simulink model "middle_ear_filter"  (R2020b)
settings: Solver=FixedStepDiscrete  StartTime=0.0  StopTime=stopTime  RelTol=1e-3
InitFcn:
  | initCallback
StopFcn:
  | stopCallback
values from neighbouring files (symbols this model uses):
  MEcoeffs = [m14*m11 m15*m11 m16*m11 1 m12*m11 m13*m11; m24*m21 m25*m21 m26*m21 1 m22*m21 m23*m21; m34*m31 m35*m31 m36*m31 1 m32*m31 m33*m31]    [mef_parameters.m]    (also in middle_ear_filter_parameter.m)
  MEscale = 1/megainmax    (= 0.5)    [mef_parameters.m]    (also in middle_ear_filter_parameter.m)
undefined symbols (not defined in the file or in its folder): mp
settings Model: Creator=Ross  LastModifiedBy=conno
settings DataIOCC: ReturnWorkspaceOutputs=off
settings OptimizationCC: BlockReduction=off  ConditionallyExecuteInputs=off  DefaultParameterBehavior=Inlined
settings DebuggingCC: ReadBeforeWriteMsg=DisableAll  WriteAfterWriteMsg=DisableAll  WriteAfterReadMsg=DisableAll  AlgebraicLoopMsg=error  MultiTaskDSMMsg=none  SingleTaskRateTransMsg=error  PregeneratedLibrarySubsystemCodeDiagnostic=none  ArithmeticOperatorsInVariantConditions=warning
settings HardwareCC: ProdBitPerPointer=32  ProdBitPerSizeT=32  ProdBitPerPtrDiffT=32  ProdLargestAtomicFloat=None  ProdIntDivRoundTo=Undefined  ProdEndianess=Unspecified  ProdWordSize=32  ProdHWDeviceType=ASIC/FPGA->ASIC/FPGA  TargetBitPerPointer=64  TargetBitPerSizeT=64  TargetBitPerPtrDiffT=64  TargetLongLongMode=on  TargetIntDivRoundTo=Zero  TargetEndianess=LittleEndian  TargetWordSize=64  TargetHWDeviceType=Custom Processor->MATLAB Host Computer  ProdEqTarget=off
settings ModelReferenceCC: UpdateModelReferenceTargets=IfOutOfDate
settings SFSimCC: SFSimEcho=off  SimUseLocalCustomCode=off  CustomCodeUndefinedFunction=UseInterfaceOnly
settings RTWCC: RTWUseLocalCustomCode=off

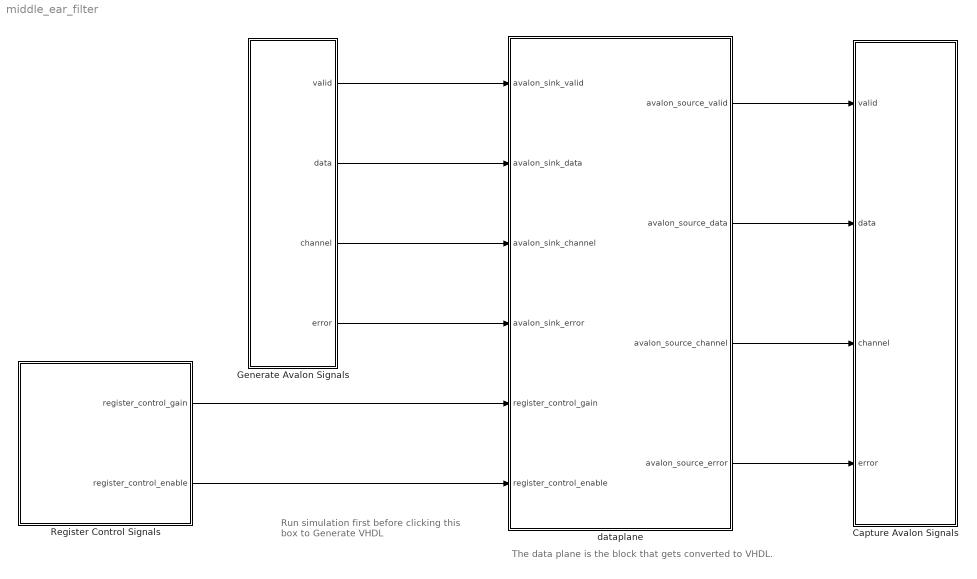
== system middle_ear_filter ==
  note: The data plane is the block that gets converted to VHDL.
  note: Run simulation first
      | before clicking this box to
      | Generate VHDL
  Capture Avalon Signals : Subsystem
  Generate Avalon Signals : Subsystem
  Register Control Signals : Subsystem
  dataplane : Subsystem  TreatAsAtomicUnit=on
  wires:
  Generate Avalon Signals/2(data) -> dataplane/2(avalon_sink_data)
  Generate Avalon Signals/1(valid) -> dataplane/1(avalon_sink_valid)
  Generate Avalon Signals/3(channel) -> dataplane/3(avalon_sink_channel)
  Generate Avalon Signals/4(error) -> dataplane/4(avalon_sink_error)
  dataplane/2(avalon_source_data) -> Capture Avalon Signals/2(data)
  dataplane/1(avalon_source_valid) -> Capture Avalon Signals/1(valid)
  dataplane/3(avalon_source_channel) -> Capture Avalon Signals/3(channel)
  dataplane/4(avalon_source_error) -> Capture Avalon Signals/4(error)
  Register Control Signals/1(register_control_gain) -> dataplane/5(register_control_gain)
  Register Control Signals/2(register_control_enable) -> dataplane/6(register_control_enable)

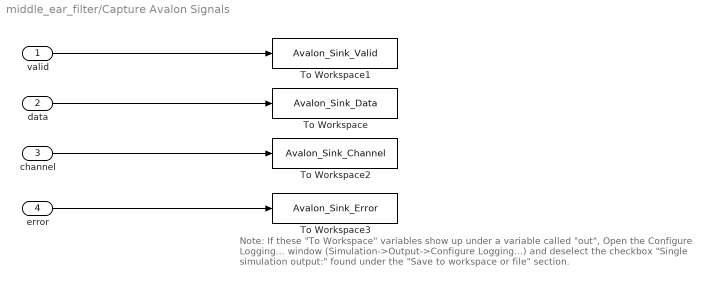
== system middle_ear_filter/Capture Avalon Signals ==
  note: Note:  If these "To Workspace" variables show up under a variable called "out",
      | Open the Configure Logging... window (Simulation->Output->Configure Logging...)
      | and deselect the checkbox "Single simulation output:" found under the "Save to workspace or file" section.
  valid : Inport
  data : Inport  Port=2
  channel : Inport  Port=3
  error : Inport  Port=4
  To Workspace : ToWorkspace  VariableName=Avalon_Sink_Data  SaveFormat=Timeseries  SampleTime=-1
  To Workspace1 : ToWorkspace  VariableName=Avalon_Sink_Valid  SaveFormat=Timeseries  SampleTime=-1
  To Workspace2 : ToWorkspace  VariableName=Avalon_Sink_Channel  SaveFormat=Timeseries  SampleTime=-1
  To Workspace3 : ToWorkspace  VariableName=Avalon_Sink_Error  SaveFormat=Timeseries  SampleTime=-1
  wires:
  data/1 -> To Workspace/1
  valid/1 -> To Workspace1/1
  error/1 -> To Workspace3/1
  channel/1 -> To Workspace2/1

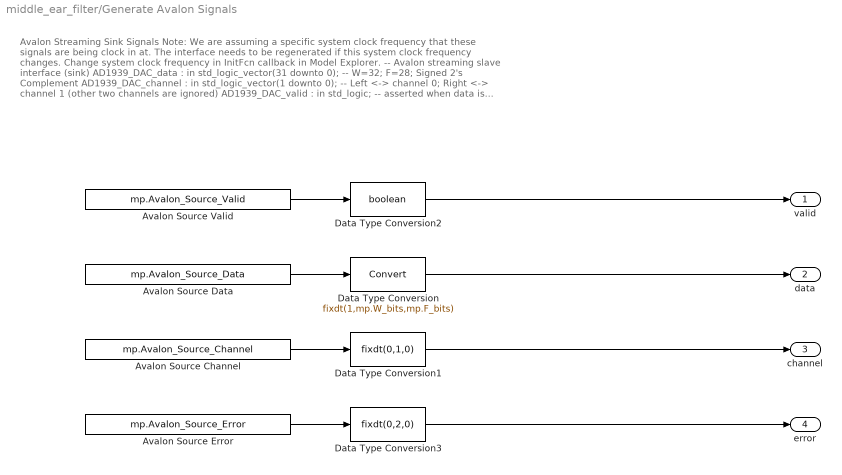
== system middle_ear_filter/Generate Avalon Signals ==
  note: Avalon Streaming Sink Signals
      | Note: We are assuming a specific system clock frequency that these signals are being clock in at.
      | The interface needs to be regenerated if this system clock frequency changes. Change system clock frequency in InitFcn callback in Model Explorer.
      |
      | -- Avalon streaming slave interface (sink)
      | AD1939_DAC_data : in std_logic_vector(31 downto 0); -- W=32; F=28; Signed 2's Complement
      | AD1939_DAC_channel : in std_logic_vector(1 downto 0); -- Left <-> channel 0; Right <-> channel 1 (other two channels are ignored)
      | AD1939_DAC_valid : in std_logic; -- asserted when data is valid
      | AD1939_DAC_error : in std_logic_vector(1 downto 0) -- error channel is ignored, assumed to be error free at this point
      |
      | For more information on the data-channel-valid protocol, s ee chapter 5 in Intel's Avalon Interfaced Specification (p. 40) at https://www.intel.com/content/dam/www/programmable/us/en/pdfs/literature/manual/mnl_avalon_spec.pdf
  Avalon Source Channel : FromWorkspace  VariableName=mp.Avalon_Source_Channel  OutDataTypeStr=double  SampleTime=mp.Ts_sim
  "Avalon Source Data " : FromWorkspace  VariableName=mp.Avalon_Source_Data  OutDataTypeStr=double  SampleTime=mp.Ts_sim
  Avalon Source Error : FromWorkspace  VariableName=mp.Avalon_Source_Error  OutDataTypeStr=double  SampleTime=mp.Ts_sim
  Avalon Source Valid : FromWorkspace  VariableName=mp.Avalon_Source_Valid  OutDataTypeStr=double  SampleTime=mp.Ts_sim
  Data Type Conversion : DataTypeConversion  OutDataTypeStr=fixdt(1,mp.W_bits,mp.F_bits)
  Data Type Conversion1 : DataTypeConversion  OutDataTypeStr=fixdt(0,1,0)
  Data Type Conversion2 : DataTypeConversion  OutDataTypeStr=boolean
  Data Type Conversion3 : DataTypeConversion  OutDataTypeStr=fixdt(0,2,0)
  valid : Outport  VectorParamsAs1DForOutWhenUnconnected=off
  data : Outport  Port=2  VectorParamsAs1DForOutWhenUnconnected=off
  channel : Outport  Port=3  VectorParamsAs1DForOutWhenUnconnected=off
  error : Outport  Port=4  VectorParamsAs1DForOutWhenUnconnected=off
  wires:
  Data Type Conversion1/1 -> channel/1
  Data Type Conversion2/1 -> valid/1
  Avalon Source Error/1 -> Data Type Conversion3/1
  Data Type Conversion/1 -> data/1
  Avalon Source Valid/1 -> Data Type Conversion2/1
  Data Type Conversion3/1 -> error/1
  Avalon Source Channel/1 -> Data Type Conversion1/1
  "Avalon Source Data "/1 -> Data Type Conversion/1

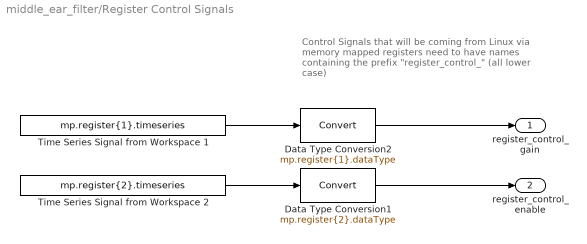
== system middle_ear_filter/Register Control Signals ==
  note: Control Signals that will be coming from Linux via
      | memory mapped registers need to have names
      | containing the prefix "register_control_"
      | (all lower case)
  Data Type Conversion1 : DataTypeConversion  OutDataTypeStr=mp.register{2}.dataType
  Data Type Conversion2 : DataTypeConversion  OutDataTypeStr=mp.register{1}.dataType
  Time Series Signal from Workspace 1 : FromWorkspace  VariableName=mp.register{1}.timeseries  OutDataTypeStr=double  SampleTime=mp.Ts_sim
  Time Series Signal from Workspace 2 : FromWorkspace  VariableName=mp.register{2}.timeseries  OutDataTypeStr=double  SampleTime=mp.Ts_sim
  register_control_gain : Outport  VectorParamsAs1DForOutWhenUnconnected=off
  register_control_enable : Outport  Port=2  VectorParamsAs1DForOutWhenUnconnected=off
  wires:
  Time Series Signal from Workspace 1/1 -> Data Type Conversion2/1
  Data Type Conversion2/1 -> register_control_gain/1
  Data Type Conversion1/1 -> register_control_enable/1
  Time Series Signal from Workspace 2/1 -> Data Type Conversion1/1

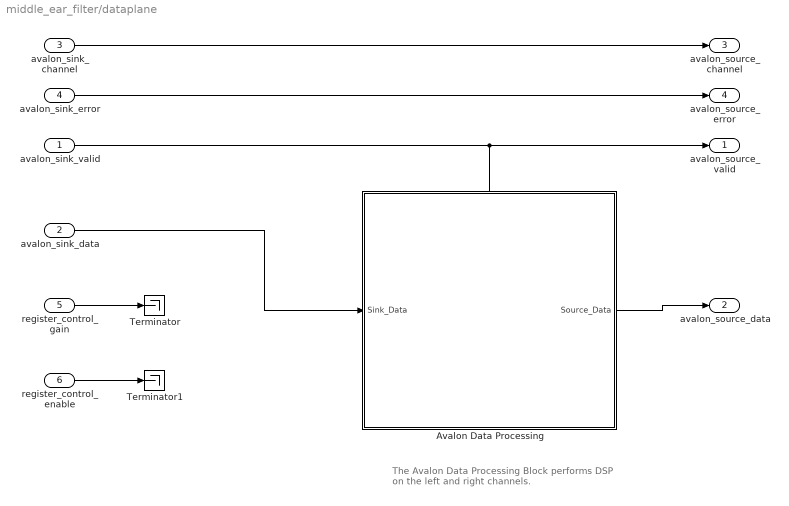
== system middle_ear_filter/dataplane ==
  note: The Avalon Data Processing Block
      | performs DSP on the left and right channels.
  avalon_sink_valid : Inport
  avalon_sink_data : Inport  Port=2
  avalon_sink_channel : Inport  Port=3
  avalon_sink_error : Inport  Port=4
  register_control_gain : Inport  Port=5
  register_control_enable : Inport  Port=6
  Avalon Data Processing : Subsystem  TreatAsAtomicUnit=on
  Terminator : Terminator
  Terminator1 : Terminator
  avalon_source_valid : Outport  VectorParamsAs1DForOutWhenUnconnected=off
  avalon_source_data : Outport  Port=2  VectorParamsAs1DForOutWhenUnconnected=off
  avalon_source_channel : Outport  Port=3  VectorParamsAs1DForOutWhenUnconnected=off
  avalon_source_error : Outport  Port=4  VectorParamsAs1DForOutWhenUnconnected=off
  wires:
  avalon_sink_error/1 -> avalon_source_error/1
  avalon_sink_valid/1 -> avalon_source_valid/1
  avalon_sink_data/1 -> Avalon Data Processing/1(Sink_Data)
  register_control_gain/1 -> Terminator/1
  Avalon Data Processing/1(Source_Data) -> avalon_source_data/1
  avalon_sink_channel/1 -> avalon_source_channel/1
  register_control_enable/1 -> Terminator1/1

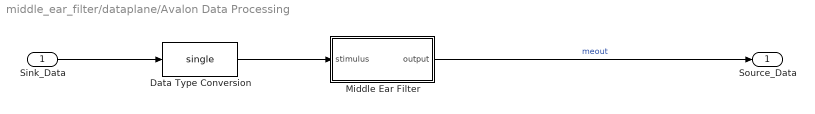
== system middle_ear_filter/dataplane/Avalon Data Processing ==
  Sink_Data : Inport
  Data Type Conversion : DataTypeConversion  OutDataTypeStr=single
  Middle Ear Filter : Subsystem
  Source_Data : Outport  InitialOutput=0  VectorParamsAs1DForOutWhenUnconnected=off
  wires:
  Sink_Data/1 -> Data Type Conversion/1
  Middle Ear Filter/1(output) -> Source_Data/1  "meout"
  Data Type Conversion/1 -> Middle Ear Filter/1(stimulus)

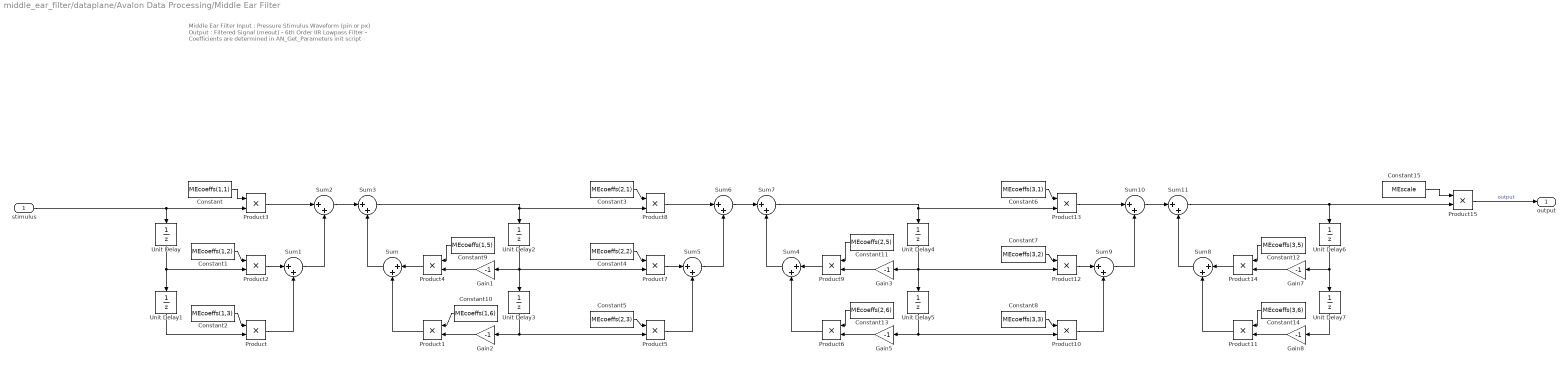
== system middle_ear_filter/dataplane/Avalon Data Processing/Middle Ear Filter ==
  note: Middle Ear Filter
      |
      | Input : Pressure Stimulus Waveform (pin or px)
      |
      | Output : Filtered Signal (meout)
      |
      | - 6th Order IIR Lowpass Filter
      |
      | - Coefficients are determined in AN_Get_Parameters init script
  stimulus : Inport  OutDataTypeStr=single  PortDimensions=1  SampleTime=[2.0833333333333333e-05,0]
  Constant : Constant  Value=MEcoeffs(1,1)  OutDataTypeStr=single  SampleTime=-1
  Constant1 : Constant  Value=MEcoeffs(1,2)  OutDataTypeStr=single  SampleTime=-1
  Constant10 : Constant  Value=MEcoeffs(1,6)  OutDataTypeStr=single  SampleTime=-1
  Constant11 : Constant  Value=MEcoeffs(2,5)  OutDataTypeStr=single  SampleTime=-1
  Constant12 : Constant  Value=MEcoeffs(3,5)  OutDataTypeStr=single  SampleTime=-1
  Constant13 : Constant  Value=MEcoeffs(2,6)  OutDataTypeStr=single  SampleTime=-1
  Constant14 : Constant  Value=MEcoeffs(3,6)  OutDataTypeStr=single  SampleTime=-1
  Constant15 : Constant  Value=MEscale  OutDataTypeStr=single  SampleTime=-1
  Constant2 : Constant  Value=MEcoeffs(1,3)  OutDataTypeStr=single  SampleTime=-1
  Constant3 : Constant  Value=MEcoeffs(2,1)  OutDataTypeStr=single  SampleTime=-1
  Constant4 : Constant  Value=MEcoeffs(2,2)  OutDataTypeStr=single  SampleTime=-1
  Constant5 : Constant  Value=MEcoeffs(2,3)  OutDataTypeStr=single  SampleTime=-1
  Constant6 : Constant  Value=MEcoeffs(3,1)  OutDataTypeStr=single  SampleTime=-1
  Constant7 : Constant  Value=MEcoeffs(3,2)  OutDataTypeStr=single  SampleTime=-1
  Constant8 : Constant  Value=MEcoeffs(3,3)  OutDataTypeStr=single  SampleTime=-1
  Constant9 : Constant  Value=MEcoeffs(1,5)  OutDataTypeStr=single  SampleTime=-1
  Gain{1..3,5,7..8} (6 alike) : Gain  Gain=-1
  Product{,1..15} (16 alike) : Product
  Sum{,1..11} (12 alike) : Sum  Inputs=|++
  Unit Delay{,1..7} (8 alike) : UnitDelay  SampleTime=-1  HasFrameUpgradeWarning=on
  output : Outport  OutDataTypeStr=single  PortDimensions=1  SampleTime=[2.0833333333333333e-05,0]  VectorParamsAs1DForOutWhenUnconnected=off
  wires:
  Product9/1 -> Sum4/1
  Sum9/1 -> Sum10/2
  Gain1/1 -> Product4/2
  Constant3/1 -> Product8/1
  Gain3/1 -> Product9/2
  Product12/1 -> Sum9/1
  Unit Delay4/1 -> Gain3/1, Unit Delay5/1, Product12/2
  Gain5/1 -> Product6/2
  Constant15/1 -> Product15/1
  Sum11/1 -> Unit Delay6/1, Product15/2
  Unit Delay/1 -> Product2/2, Unit Delay1/1
  Sum/1 -> Sum3/2
  Sum10/1 -> Sum11/1
  stimulus/1 -> Unit Delay/1, Product3/2
  Product/1 -> Sum1/2
  Constant10/1 -> Product1/1
  Sum1/1 -> Sum2/2
  Product5/1 -> Sum5/2
  Constant9/1 -> Product4/1
  Unit Delay3/1 -> Gain2/1, Product5/2
  Product8/1 -> Sum6/1
  Gain8/1 -> Product11/2
  Unit Delay6/1 -> Gain7/1, Unit Delay7/1
  Product13/1 -> Sum10/1
  Product1/1 -> Sum/2
  Unit Delay2/1 -> Gain1/1, Unit Delay3/1, Product7/2
  Constant5/1 -> Product5/1
  Product4/1 -> Sum/1
  Constant/1 -> Product3/1
  Sum6/1 -> Sum7/1
  Sum7/1 -> Unit Delay4/1, Product13/2
  Product2/1 -> Sum1/1
  Product10/1 -> Sum9/2
  Constant7/1 -> Product12/1
  Sum5/1 -> Sum6/2
  Constant6/1 -> Product13/1
  Sum3/1 -> Unit Delay2/1, Product8/2
  Sum2/1 -> Sum3/1
  Gain2/1 -> Product1/2
  Unit Delay7/1 -> Gain8/1
  Product11/1 -> Sum8/2
  Constant14/1 -> Product11/1
  Product7/1 -> Sum5/1
  Sum4/1 -> Sum7/2
  Unit Delay1/1 -> Product/2
  Constant12/1 -> Product14/1
  Constant2/1 -> Product/1
  Constant1/1 -> Product2/1
  Product3/1 -> Sum2/1
  Sum8/1 -> Sum11/2
  Product6/1 -> Sum4/2
  Constant4/1 -> Product7/1
  Unit Delay5/1 -> Gain5/1, Product10/2
  Constant13/1 -> Product6/1
  Constant11/1 -> Product9/1
  Product14/1 -> Sum8/1
  Product15/1 -> output/1  "output"
  Constant8/1 -> Product10/1
  Gain7/1 -> Product14/2
